simulink subsystem "quat_dyn_body_w_wheels"  (R2022a)
settings: Solver=VariableStepAuto  StartTime=0.0  StopTime=10.0  RelTol=1e-3
libraries: matrix_library x1, aerolibutil x1
settings Model: Creator=samuel  LastModifiedBy=samuel

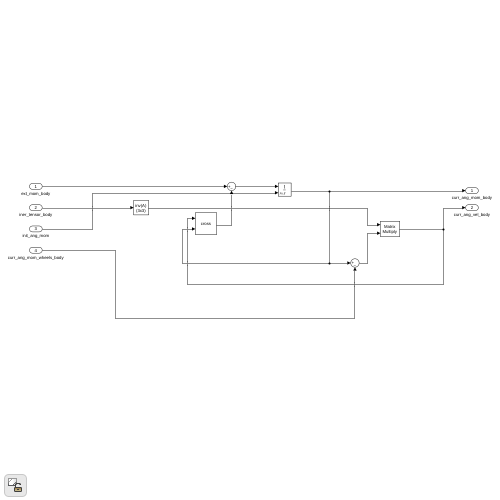
[thumbnail: Simulink's stored preview of the top-level diagram]
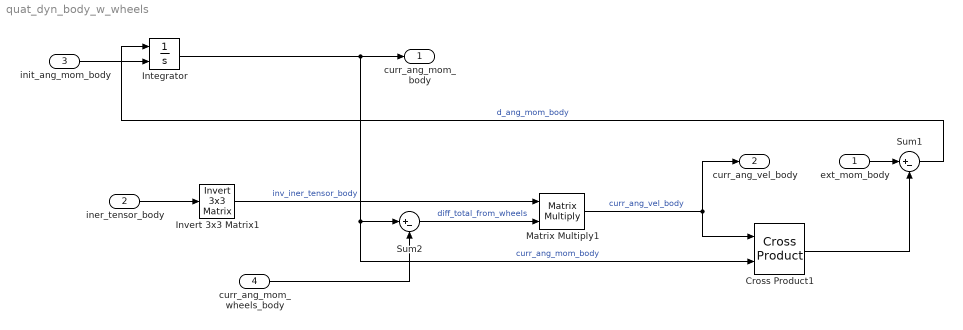
== system quat_dyn_body_w_wheels ==
  ext_mom_body : Inport
  iner_tensor_body : Inport  Port=2
  init_ang_mom_body : Inport  Port=3
  curr_ang_mom_wheels_body : Inport  Port=4
  Cross Product1 : matrix_library/Cross Product
      settings: SourceProductBaseCode=SL
  Integrator : Integrator  InitialConditionSource=external
  Invert 3x3 Matrix1 : aerolibutil/Invert  3x3 Matrix
  Matrix Multiply1 : Product  Multiplication=Matrix(*)
  Sum1 : Sum  Inputs=|+-
  Sum2 : Sum  Inputs=|+-
  curr_ang_mom_body : Outport
  curr_ang_vel_body : Outport  Port=2
  wires:
  ext_mom_body/1 -> Sum1/1
  Invert 3x3 Matrix1/1 -> Matrix Multiply1/1  "inv_iner_tensor_body"
  Sum1/1 -> Integrator/1  "d_ang_mom_body"
  Sum2/1 -> Matrix Multiply1/2  "diff_total_from_wheels"
  Cross Product1/1 -> Sum1/2
  init_ang_mom_body/1 -> Integrator/2
  Integrator/1 -> Cross Product1/2, Sum2/1, curr_ang_mom_body/1  "curr_ang_mom_body"
  curr_ang_mom_wheels_body/1 -> Sum2/2
  iner_tensor_body/1 -> Invert 3x3 Matrix1/1
  Matrix Multiply1/1 -> Cross Product1/1, curr_ang_vel_body/1  "curr_ang_vel_body"
